simulink model "untitled"  (R2016a)
settings: Solver=VariableStepAuto  StartTime=0.0  StopTime=10.0  RelTol=1e-3
settings Model: Creator=EDU Student  LastModifiedBy=EDU Student

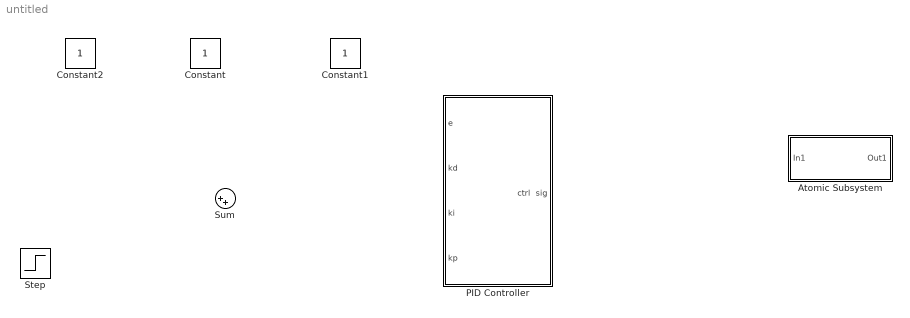
== system untitled ==
  Atomic Subsystem : Subsystem  TreatAsAtomicUnit=on
  Constant : Constant
  Constant1 : Constant
  Constant2 : Constant
  "PID Controller " : Subsystem  TreatAsAtomicUnit=on
  Step : Step  SampleTime=0
  Sum : Sum  Inputs=|++

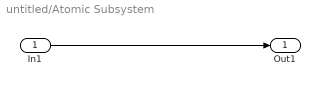
== system untitled/Atomic Subsystem ==
  In1 : Inport
  Out1 : Outport
  wires:
  In1/1 -> Out1/1

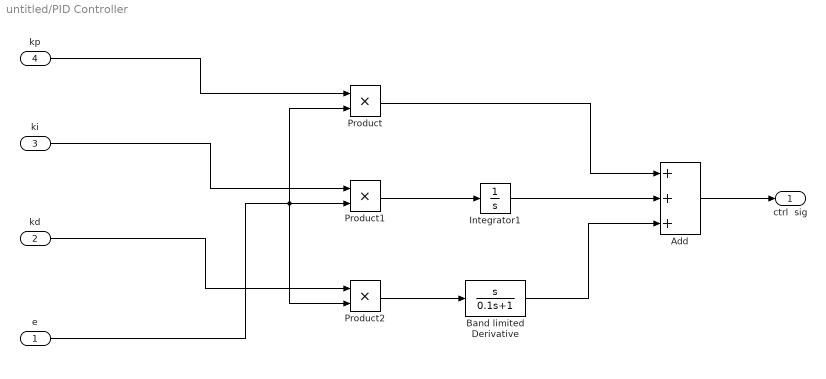
== system untitled/PID Controller  ==
  e : Inport
  kd : Inport  Port=2
  ki : Inport  Port=3
  kp : Inport  Port=4
  Add : Sum  Inputs=+++
  Band limited Derivative : TransferFcn  Numerator=[1 0]  Denominator=[0 0.1 1]
  Integrator1 : Integrator
  Product : Product
  Product1 : Product
  Product2 : Product
  ctrl  sig : Outport
  wires:
  kp/1 -> Product/1
  kd/1 -> Product2/1
  ki/1 -> Product1/1
  e/1 -> Product/2, Product2/2, Product1/2
  Product1/1 -> Integrator1/1
  Integrator1/1 -> Add/2
  Band limited Derivative/1 -> Add/3
  Product/1 -> Add/1
  Product2/1 -> Band limited Derivative/1
  Add/1 -> ctrl  sig/1
